simulink model "scara"  (R2020a)
settings: Solver=VariableStepAuto  StartTime=0.0  StopTime=10.0  RelTol=1e-3  EnableMultiTasking=on
values from neighbouring files (symbols this model uses):
  a2 = 180    [scara_data.m]
  a3 = 0    [scara_data.m]
  a4 = 0    [scara_data.m]
  alpha2 = 180    [scara_data.m]
  alpha3 = 0    [scara_data.m]
  alpha4 = 0    [scara_data.m]
  ceta2 = 0    [scara_data.m]
  ceta3 = 0    [scara_data.m]
  ceta4 = 0    [scara_data.m]
  d2 = 0    [scara_data.m]
  d3 = 100    [scara_data.m]
  d4 = 77    [scara_data.m]
undefined symbols (not defined in the file or in its folder): a1, alpha1, ceta1, d1
settings Model: Creator=Amr  LastModifiedBy=Amr
settings DataIOCC: ReturnWorkspaceOutputs=off
settings OptimizationCC: LifeSpan=inf
settings DebuggingCC: SFUnexpectedBacktrackingDiag=warning  SFNoUnconditionalDefaultTransitionDiag=warning  ArithmeticOperatorsInVariantConditions=warning
settings SFSimCC: SimUseLocalCustomCode=off  CustomCodeUndefinedFunction=UseInterfaceOnly
settings RTWCC: RTWUseLocalCustomCode=off
settings CodeAppCC: StateflowObjectComments=on
settings GRTTargetCC: TargetLangStandard=C89/C90 (ANSI)
settings ConfigComp: CovMetricSettings=dw  CovHtmlReporting=on  CovSaveCumulativeToWorkspaceVar=on  CovSaveSingleToWorkspaceVar=on  CovExternalEMLEnable=off

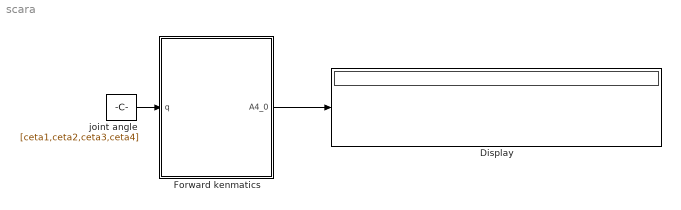
== system scara ==
  Display : Display
      settings: Format=bank
  Forward kenmatics : Subsystem
  joint angle : Constant  Value=[ceta1,ceta2,ceta3,ceta4]
  wires:
  Forward kenmatics/1(A4_0) -> Display/1
  joint angle/1 -> Forward kenmatics/1(q)

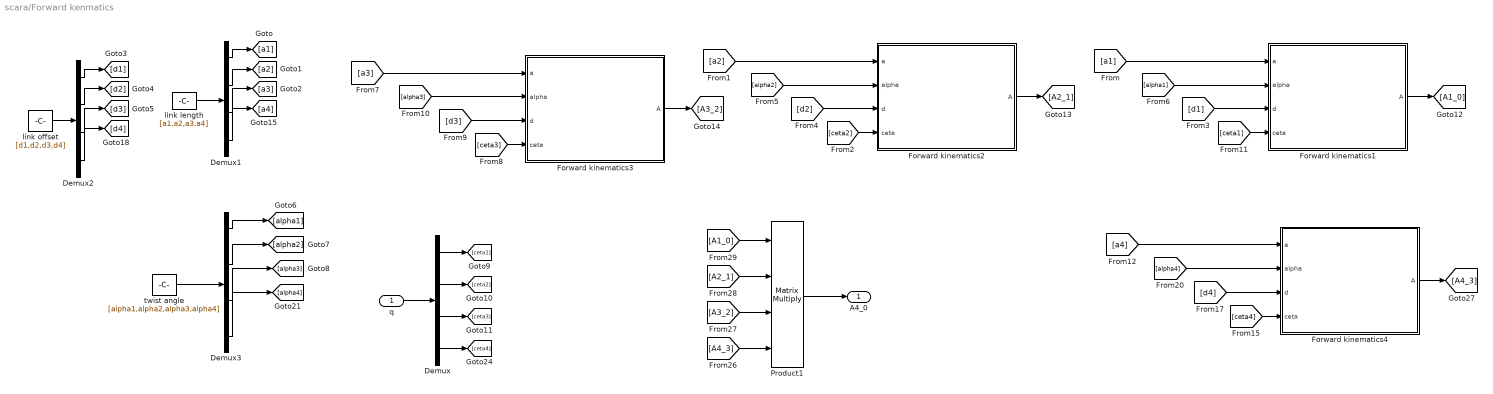
== system scara/Forward kenmatics ==
  q : Inport
  " Forward kinematics1" : MATLAB Function  TreatAsAtomicUnit=on
  " Forward kinematics2" : MATLAB Function  TreatAsAtomicUnit=on
  " Forward kinematics3" : MATLAB Function  TreatAsAtomicUnit=on
  " Forward kinematics4" : MATLAB Function  TreatAsAtomicUnit=on
  Demux{,1..3} (4 alike) : Demux
  Product1 : Product  Inputs=4  Multiplication=Matrix(*)
  link length : Constant  Value=[a1,a2,a3,a4]
  link offset : Constant  Value=[d1,d2,d3,d4]
  twist angle : Constant  Value=[alpha1,alpha2,alpha3,alpha4]
  A4_0 : Outport
  wires:
  Demux2/4 -> [d4]
  " Forward kinematics3"/1(A) -> [A3_2]
  Demux1/4 -> [a4]
  Demux/4 -> [ceta4]
  " Forward kinematics1"/1(A) -> [A1_0]
  [d2] -> " Forward kinematics2"/3(d)
  [a2] -> " Forward kinematics2"/1(a)
  [alpha2] -> " Forward kinematics2"/2(alpha)
  [ceta2] -> " Forward kinematics2"/4(ceta)
  [ceta4] -> " Forward kinematics4"/4(ceta)
  [alpha4] -> " Forward kinematics4"/2(alpha)
  [a4] -> " Forward kinematics4"/1(a)
  [d4] -> " Forward kinematics4"/3(d)
  " Forward kinematics4"/1(A) -> [A4_3]
  " Forward kinematics2"/1(A) -> [A2_1]
  Demux3/4 -> [alpha4]
  [d3] -> " Forward kinematics3"/3(d)
  [ceta3] -> " Forward kinematics3"/4(ceta)
  [a3] -> " Forward kinematics3"/1(a)
  [alpha3] -> " Forward kinematics3"/2(alpha)
  Demux1/1 -> [a1]
  Demux1/2 -> [a2]
  q/1 -> Demux/1
  Demux1/3 -> [a3]
  link offset/1 -> Demux2/1
  Demux2/1 -> [d1]
  Product1/1 -> A4_0/1
  Demux/1 -> [ceta1]
  [ceta1] -> " Forward kinematics1"/4(ceta)
  Demux3/1 -> [alpha1]
  Demux2/3 -> [d3]
  [a1] -> " Forward kinematics1"/1(a)
  Demux/2 -> [ceta2]
  Demux/3 -> [ceta3]
  Demux2/2 -> [d2]
  [d1] -> " Forward kinematics1"/3(d)
  link length/1 -> Demux1/1
  Demux3/2 -> [alpha2]
  [alpha1] -> " Forward kinematics1"/2(alpha)
  Demux3/3 -> [alpha3]
  [A3_2] -> Product1/3
  [A1_0] -> Product1/1
  [A2_1] -> Product1/2
  [A4_3] -> Product1/4
  twist angle/1 -> Demux3/1

== matlab function scara/Forward kenmatics/ Forward kinematics2 ==
  data: a input; alpha input; A output; d input; ceta input

function  A=fk_transformation_matrix(a,alpha,d,ceta )


A=[cosd(ceta) , (-1*sind(ceta)*cosd(alpha)) , (sind(ceta)*sind(alpha)) , (a*cosd(ceta)) ;...........................
    sind(ceta) , (cosd(ceta)*cosd(alpha)) ,(-1*cosd(ceta)*sind(alpha)) , (a*sind(ceta)) ;............................
    0 , sind(alpha) , cosd(alpha) , d ;..................................................................................
    0,0,0,1];

== matlab function scara/Forward kenmatics/ Forward kinematics3 ==
  data: a input; alpha input; A output; d input; ceta input

function  A=fk_transformation_matrix(a,alpha,d,ceta )


A=[cosd(ceta) , (-1*sind(ceta)*cosd(alpha)) , (sind(ceta)*sind(alpha)) , (a*cosd(ceta)) ;...........................
    sind(ceta) , (cosd(ceta)*cosd(alpha)) ,(-1*cosd(ceta)*sind(alpha)) , (a*sind(ceta)) ;............................
    0 , sind(alpha) , cosd(alpha) , d ;..................................................................................
    0,0,0,1];

== matlab function scara/Forward kenmatics/ Forward kinematics4 ==
  data: a input; alpha input; A output; d input; ceta input

function  A=fk_transformation_matrix(a,alpha,d,ceta )


A=[cosd(ceta) , (-1*sind(ceta)*cosd(alpha)) , (sind(ceta)*sind(alpha)) , (a*cosd(ceta)) ;...........................
    sind(ceta) , (cosd(ceta)*cosd(alpha)) ,(-1*cosd(ceta)*sind(alpha)) , (a*sind(ceta)) ;............................
    0 , sind(alpha) , cosd(alpha) , d ;..................................................................................
    0,0,0,1];

== matlab function scara/Forward kenmatics/ Forward kinematics1 ==
  data: a input; alpha input; A output; d input; ceta input

function  A=fk_transformation_matrix(a,alpha,d,ceta )


A=[cosd(ceta) , (-1*sind(ceta)*cosd(alpha)) , (sind(ceta)*sind(alpha)) , (a*cosd(ceta)) ;...........................
    sind(ceta) , (cosd(ceta)*cosd(alpha)) ,(-1*cosd(ceta)*sind(alpha)) , (a*sind(ceta)) ;............................
    0 , sind(alpha) , cosd(alpha) , d ;..................................................................................
    0,0,0,1];
